simulink model "ModelPendulumObserver"  (R2024a)
settings: Solver=VariableStepAuto  StartTime=0.0  StopTime=T_sim  RelTol=1e-3
undefined symbols (not defined in the file): L_gain, ssmodel_C, ssmodel_discrete_A, ssmodel_discrete_B, Ts_ensaio
settings Model: Creator=Douglas  LastModifiedBy=Douglas

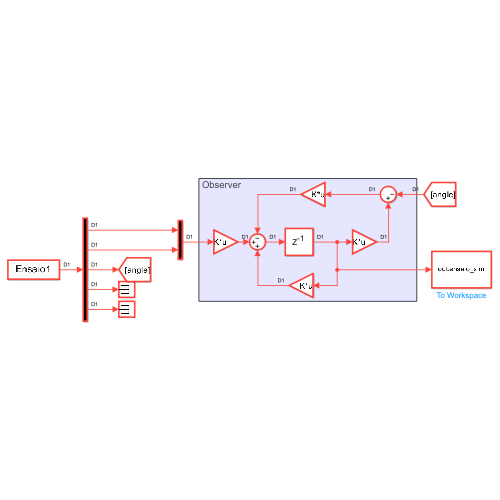
[thumbnail: Simulink's stored preview of the top-level diagram]
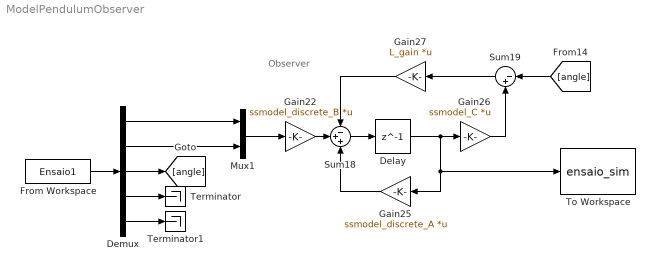
== system ModelPendulumObserver ==
  note: Observer
  Delay : Delay  DelayLength=1
  Demux : Demux  Outputs=5
  From Workspace : FromWorkspace  VariableName=Ensaio1  SampleTime=Ts_ensaio
  Gain22 : Gain  Gain=ssmodel_discrete_B  Multiplication=Matrix(K*u)
  Gain25 : Gain  Gain=ssmodel_discrete_A  Multiplication=Matrix(K*u)
  Gain26 : Gain  Gain=ssmodel_C  Multiplication=Matrix(K*u)
  Gain27 : Gain  Gain=L_gain  Multiplication=Matrix(K*u)
  Mux1 : Mux  Inputs=2
  Sum18 : Sum  Inputs=-++
  Sum19 : Sum  Inputs=|-+
  Terminator : Terminator
  Terminator1 : Terminator
  To Workspace : ToWorkspace  VariableName=ensaio_sim  SaveFormat=Structure  SampleTime=Ts_ensaio
  wires:
  From Workspace/1 -> Demux/1
  Demux/1 -> Mux1/1
  Demux/2 -> Mux1/2
  Demux/4 -> Terminator/1
  Demux/5 -> Terminator1/1
  Demux/3 -> [angle]
  Delay/1 -> Gain26/1, To Workspace/1, Gain25/1
  Sum19/1 -> Gain27/1
  Sum18/1 -> Delay/1
  Gain27/1 -> Sum18/1
  [angle] -> Sum19/1
  Gain22/1 -> Sum18/2
  Gain25/1 -> Sum18/3
  Gain26/1 -> Sum19/2
  Mux1/1 -> Gain22/1
